simulink model "Test_Demultiplexer"  (Simulink 8.1)
settings: Solver=ode45  StartTime=0.0  StopTime=10.0  RelTol=1e-3
libraries: Computer_Library x6, commutil2 x4
settings Model: Creator=N  LastModifiedBy=uzivatel
settings DataIOCC: LimitDataPoints=off  SignalLoggingSaveFormat=Dataset
settings OptimizationCC: ExpressionDepthLimit=128
settings DebuggingCC: UnderspecifiedInitializationDetection=Simplified  MergeDetectMultiDrivingBlocksExec=error  SolverPrmCheckMsg=none  FcnCallInpInsideContextMsg=EnableAllAsError  FrameProcessingCompatibilityMsg=error  StateNameClashWarn=none
settings HardwareCC: ProdBitPerPointer=64  ProdLargestAtomicFloat=Float  ProdIntDivRoundTo=Zero  ProdEndianess=LittleEndian  ProdHWDeviceType=Intel->x86-64 (Windows64)
settings ModelReferenceCC: PropagateSignalLabelsOutOfModel=on
settings GRTTargetCC: CodeReplacementLibrary=None  CombineOutputUpdateFcns=on  CPPClassGenCompliant=on  GRTInterface=off

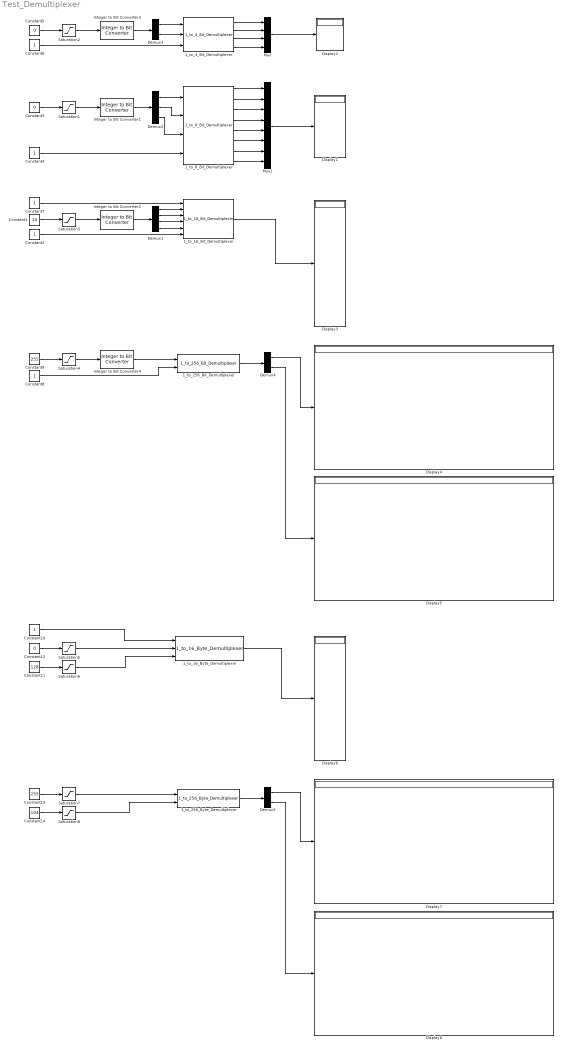
== system Test_Demultiplexer ==
  1_to_16_Bit_Demultiplexer : Computer_Library/Demultiplexers/1_to_16_Bit_Demultiplexer
  1_to_16_Byte_Demultiplexer : Computer_Library/Demultiplexers/1_to_16_Byte_Demultiplexer
  1_to_256_Bit_Demultiplexer : Computer_Library/Demultiplexers/1_to_256_Bit_Demultiplexer
  1_to_256_Byte_Demultiplexer : Computer_Library/Demultiplexers/1_to_256_Byte_Demultiplexer
  1_to_4_Bit_Demultiplexer : Computer_Library/Demultiplexers/1_to_4_Bit_Demultiplexer
  1_to_8_Bit_Demultiplexer : Computer_Library/Demultiplexers/1_to_8_Bit_Demultiplexer
  Constant1 : Constant  Value=14
  Constant{2,4,6..8,10} (6 alike) : Constant
  Constant11 : Constant  Value=128
  Constant12 : Constant  Value=0
  Constant13 : Constant  Value=255
  Constant14 : Constant  Value=104
  Constant3 : Constant  Value=0
  Constant5 : Constant  Value=0
  Constant9 : Constant  Value=255
  Demux1 : Demux
  Demux2 : Demux  Outputs=3
  Demux3 : Demux  Outputs=2
  Demux4 : Demux  Outputs=2
  Demux5 : Demux  Outputs=2
  Display{1..8} (8 alike) : Display
  Integer to Bit Converter1 : commutil2/Integer to Bit Converter  nbits=3  signedInputValues=Unsigned  bitOrder=MSB first  outDtype=int8
  Integer to Bit Converter2 : commutil2/Integer to Bit Converter  nbits=4  signedInputValues=Unsigned  bitOrder=MSB first  outDtype=int8
  Integer to Bit Converter3 : commutil2/Integer to Bit Converter  nbits=2  signedInputValues=Unsigned  bitOrder=MSB first  outDtype=int8
  Integer to Bit Converter4 : commutil2/Integer to Bit Converter  nbits=8  signedInputValues=Unsigned  bitOrder=MSB first  outDtype=uint8
  Mux : Mux
  Mux1 : Mux  Inputs=8
  Saturation1 : Saturate  UpperLimit=7  LowerLimit=0
  Saturation2 : Saturate  UpperLimit=3  LowerLimit=0
  Saturation3 : Saturate  UpperLimit=15  LowerLimit=0
  Saturation{4,6..8} (4 alike) : Saturate  UpperLimit=255  LowerLimit=0
  Saturation5 : Saturate  UpperLimit=15  LowerLimit=0
  wires:
  Demux1/1 -> 1_to_16_Bit_Demultiplexer/2
  Demux1/2 -> 1_to_16_Bit_Demultiplexer/3
  Demux1/3 -> 1_to_16_Bit_Demultiplexer/4
  Demux1/4 -> 1_to_16_Bit_Demultiplexer/5
  Integer to Bit Converter2/1 -> Demux1/1
  Constant1/1 -> Saturation3/1
  Saturation3/1 -> Integer to Bit Converter2/1
  Constant2/1 -> 1_to_16_Bit_Demultiplexer/6
  1_to_16_Bit_Demultiplexer/1 -> Display3/1
  Demux2/1 -> 1_to_8_Bit_Demultiplexer/1
  Demux2/2 -> 1_to_8_Bit_Demultiplexer/2
  Demux2/3 -> 1_to_8_Bit_Demultiplexer/3
  Integer to Bit Converter1/1 -> Demux2/1
  Constant3/1 -> Saturation1/1
  Saturation1/1 -> Integer to Bit Converter1/1
  Constant4/1 -> 1_to_8_Bit_Demultiplexer/4
  Demux3/1 -> 1_to_4_Bit_Demultiplexer/1
  Demux3/2 -> 1_to_4_Bit_Demultiplexer/2
  Integer to Bit Converter3/1 -> Demux3/1
  Constant5/1 -> Saturation2/1
  Saturation2/1 -> Integer to Bit Converter3/1
  Constant6/1 -> 1_to_4_Bit_Demultiplexer/3
  1_to_4_Bit_Demultiplexer/1 -> Mux/1
  1_to_4_Bit_Demultiplexer/2 -> Mux/2
  1_to_4_Bit_Demultiplexer/3 -> Mux/3
  1_to_4_Bit_Demultiplexer/4 -> Mux/4
  1_to_8_Bit_Demultiplexer/1 -> Mux1/1
  1_to_8_Bit_Demultiplexer/8 -> Mux1/8
  1_to_8_Bit_Demultiplexer/2 -> Mux1/2
  1_to_8_Bit_Demultiplexer/3 -> Mux1/3
  1_to_8_Bit_Demultiplexer/4 -> Mux1/4
  1_to_8_Bit_Demultiplexer/5 -> Mux1/5
  1_to_8_Bit_Demultiplexer/6 -> Mux1/6
  1_to_8_Bit_Demultiplexer/7 -> Mux1/7
  Mux1/1 -> Display1/1
  Mux/1 -> Display2/1
  Constant7/1 -> 1_to_16_Bit_Demultiplexer/1
  Constant8/1 -> 1_to_256_Bit_Demultiplexer/2
  Integer to Bit Converter4/1 -> 1_to_256_Bit_Demultiplexer/1
  Saturation4/1 -> Integer to Bit Converter4/1
  Constant9/1 -> Saturation4/1
  1_to_256_Bit_Demultiplexer/1 -> Demux4/1
  Demux4/1 -> Display4/1
  Demux4/2 -> Display5/1
  Constant10/1 -> 1_to_16_Byte_Demultiplexer/1
  Constant12/1 -> Saturation5/1
  Saturation5/1 -> 1_to_16_Byte_Demultiplexer/2
  1_to_16_Byte_Demultiplexer/1 -> Display6/1
  Constant11/1 -> Saturation6/1
  Saturation6/1 -> 1_to_16_Byte_Demultiplexer/3
  1_to_256_Byte_Demultiplexer/1 -> Demux5/1
  Demux5/1 -> Display7/1
  Demux5/2 -> Display8/1
  Constant13/1 -> Saturation7/1
  Saturation7/1 -> 1_to_256_Byte_Demultiplexer/1
  Constant14/1 -> Saturation8/1
  Saturation8/1 -> 1_to_256_Byte_Demultiplexer/2
